simulink model "Shear"  (Simulink 8.3)
settings: Solver=ode45  StartTime=0.0  StopTime=inf  RelTol=1e-3
undefined symbols (not defined in the file): gray
libraries: visionsinks x2, visiongeotforms x2, visionsources x1
settings Model: Creator=FxMain  LastModifiedBy=Vasilis
settings OptimizationCC: ExpressionDepthLimit=2147483647
settings DebuggingCC: FcnCallInpInsideContextMsg=UseLocalSettings

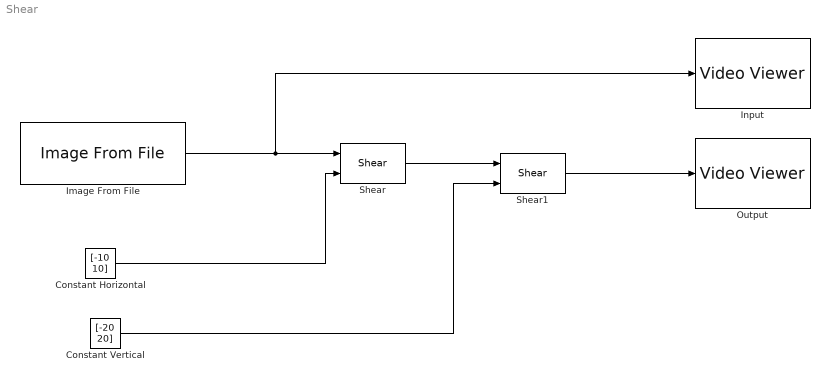
== system Shear ==
  Constant Horizontal : Constant  Value=[-10 10]  VectorParams1D=off  OutDataTypeStr=double
  Constant Vertical : Constant  Value=[-20 20]  VectorParams1D=off  OutDataTypeStr=double
  Image From File : visionsources/Image From File  Tag=vipblks_nd  FileName=peppers.png  imagePorts=One multidimensional signal  Ts=inf  ImageDataType=double  Signed=on  WordLength=16  sdImageDataType=uint(8)  FractionLengthMode=User-defined  FractionLength=15  OutPortLabels=R|G|B
  Input : visionsinks/Video Viewer  inputType=Obsolete7b  imagePorts=One multidimensional signal  useColorMap=off  colormapValue=gray(256)  specRange=off  minInputVal=0  maxInputVal=255  FigPos=[714 677 512 384]  AxisZoom=on  trueSizedOnce=on  OpenAtMdlStart=on  DefaultConfigurationName=vipscopes.VideoViewerScopeCfg
  Output : visionsinks/Video Viewer  inputType=Obsolete7b  imagePorts=One multidimensional signal  useColorMap=off  colormapValue=gray(256)  specRange=off  minInputVal=0  maxInputVal=255  FigPos=[1552 776 783 512]  AxisZoom=on  trueSizedOnce=on  OpenAtMdlStart=on  DefaultConfigurationName=vipscopes.VideoViewerScopeCfg
  Shear : visiongeotforms/Shear  direction=Horizontal  outSizeS=Full  src_shear=Input port  shear_values=[0 3]  maxShear=20  fillVal=0  interpMethod=Bilinear  prodOutputMode=Binary point scaling  prodOutputWordLength=32  prodOutputFracLength=10  roundingMode=Nearest  overflowMode=on
  Shear1 : visiongeotforms/Shear  direction=Vertical  outSizeS=Full  src_shear=Input port  shear_values=[0 3]  maxShear=40  fillVal=0  interpMethod=Bilinear  prodOutputMode=Binary point scaling  prodOutputWordLength=32  prodOutputFracLength=10  roundingMode=Nearest  overflowMode=on
  wires:
  Image From File/1 -> Input/1, Shear/1
  Constant Horizontal/1 -> Shear/2
  Shear1/1 -> Output/1
  Shear/1 -> Shear1/1
  Constant Vertical/1 -> Shear1/2
